simulink model "ParkAssist_Scenario002_cs"  (R2014b)
settings: Solver=ode5  SolverMode=SingleTasking  StartTime=0.0  StopTime=100  FixedStep=1/100  RelTol=1e-3
PreLoadFcn:
  | mbxruntime.callbacks.PreLoadFcn(bdroot);
  | check_NUTS_defined;
  | 
  | assignin('base',['model_closed_' bdroot],false);
  | addpath('../includes_AP');
PostLoadFcn:
  | mbxruntime.callbacks.PostLoadFcn(bdroot);
  | 
  | AP_PlotSpeed;
  | Sim_Stop();
InitFcn:
  | mbxruntime.callbacks.InitFcn(bdroot);
StartFcn:
  | mbxruntime.callbacks.StartFcn(bdroot);
StopFcn:
  | Sim_Stop();
  | 
  | mbxruntime.callbacks.StopFcn(bdroot);
model workspace: external: MAT-File .\ParkAssist_Scenario002_cs_hws.mat (data not in the file)
undefined symbols (not defined in the file or in its folder): mbxruntime, tabledata, warningInitialVelocity, x0
undefined symbols (not defined in the file): ParkAssist_Scenario002_cs_002fddfe84a374e6, ParkAssist_Scenario002_cs_01094a893a7092b9, ParkAssist_Scenario002_cs_02c2e05763b93088, ParkAssist_Scenario002_cs_032149ae54ddfcd1, ParkAssist_Scenario002_cs_03734bce5661314c, ParkAssist_Scenario002_cs_04091ed9282bd749, ParkAssist_Scenario002_cs_068635de1ad515a4, ParkAssist_Scenario002_cs_08968b565ab05e4d, ParkAssist_Scenario002_cs_08eaa26dcd990c9f, ParkAssist_Scenario002_cs_0a721129d3af9f72, ParkAssist_Scenario002_cs_0c5b0314074f54f3, ParkAssist_Scenario002_cs_0e48d515abeb5eec, ParkAssist_Scenario002_cs_1024d8e6ed1cbdcd, ParkAssist_Scenario002_cs_1193d522b107ebab, ParkAssist_Scenario002_cs_11dc16d46c17a7bf, ParkAssist_Scenario002_cs_13631b53806ed88f, ParkAssist_Scenario002_cs_155b57131b5ca1b3, ParkAssist_Scenario002_cs_1a68a29dae7c954c, ParkAssist_Scenario002_cs_1e925263f9fbaeb5, ParkAssist_Scenario002_cs_2102ebaddaee4634, ParkAssist_Scenario002_cs_242d7930853a635b, ParkAssist_Scenario002_cs_26123a651f74a75d, ParkAssist_Scenario002_cs_27077c166553ac4d, ParkAssist_Scenario002_cs_2775446e3f6a532e, ParkAssist_Scenario002_cs_29e1fcc85129d061, ParkAssist_Scenario002_cs_2c6c606bb8eb7e2a, ParkAssist_Scenario002_cs_2f026f6d085d63d4, ParkAssist_Scenario002_cs_2f66cf02f0c1fb02, ParkAssist_Scenario002_cs_2f7abfb8e98983ca, ParkAssist_Scenario002_cs_305144d476c37e1c, ParkAssist_Scenario002_cs_31c4862b0e1d31d2, ParkAssist_Scenario002_cs_3367812933b7aec5, ParkAssist_Scenario002_cs_338ceb4af5dab20a, ParkAssist_Scenario002_cs_359ca59699e4676c, ParkAssist_Scenario002_cs_374ade2de845ad31, ParkAssist_Scenario002_cs_390ab82ad2c54c91, ParkAssist_Scenario002_cs_391805fec31feab6, ParkAssist_Scenario002_cs_3974aed4b8055855, ParkAssist_Scenario002_cs_3a445c73fa984851, ParkAssist_Scenario002_cs_3a54967829cb62c8, ParkAssist_Scenario002_cs_3a60f4e734f7afb5, ParkAssist_Scenario002_cs_3bf2e9c0bde84b70, ParkAssist_Scenario002_cs_3c27f6f01aa99d37, ParkAssist_Scenario002_cs_3cc4b302268f6896, ParkAssist_Scenario002_cs_40419caba47c1546, ParkAssist_Scenario002_cs_42136abd911dac1d, ParkAssist_Scenario002_cs_44b760977392c607, ParkAssist_Scenario002_cs_470135ef0e52cc5f, ParkAssist_Scenario002_cs_48ebb83f5faed864, ParkAssist_Scenario002_cs_4a04bdc7976b10a4, ParkAssist_Scenario002_cs_4b414fc30cdb2355, ParkAssist_Scenario002_cs_4e3c7ad0309ae8ef, ParkAssist_Scenario002_cs_4f1cb442d755f69c, ParkAssist_Scenario002_cs_52f490d0aa621cbf, ParkAssist_Scenario002_cs_53df9d722ee02dea, ParkAssist_Scenario002_cs_5719a2c72af27d7c, ParkAssist_Scenario002_cs_575bfb9c514fb17e, ParkAssist_Scenario002_cs_588d2ca56dde3768, ParkAssist_Scenario002_cs_58ef6c537dd8a6a1, ParkAssist_Scenario002_cs_592f78d63a6470cd ... (+97)
libraries: PreScanUsefulBlocks x57, simulink x55, PreScanSimulinkLibrary x54, simulink_extras x6
(part 2 of 15)

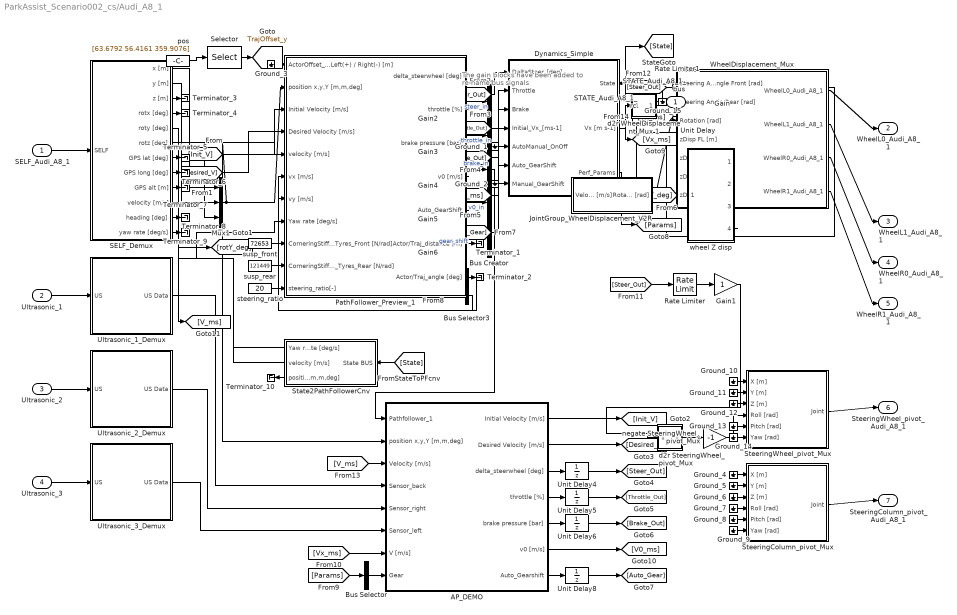
== system ParkAssist_Scenario002_cs/Audi_A8_1 ==
  note: The gain blocks have been added
      | to re-name bus signals
  SELF_Audi_A8_1 : Inport  Tag=inport/SelfPort  OutDataTypeStr=Bus: PRESCAN_SELFSENSORDATA  PortDimensions=1  SampleTime=1/100  BusOutputAsStruct=on
  Ultrasonic_1 : Inport  Tag=inport/UltraSonic  Port=2  OutDataTypeStr=Bus: PRESCAN_SCANNERSENSOR_MESSAGE  PortDimensions=1  SampleTime=1/20  BusOutputAsStruct=on
  Ultrasonic_2 : Inport  Tag=inport/UltraSonic  Port=3  OutDataTypeStr=Bus: PRESCAN_SCANNERSENSOR_MESSAGE  PortDimensions=1  SampleTime=1/20  BusOutputAsStruct=on
  Ultrasonic_3 : Inport  Tag=inport/UltraSonic  Port=4  OutDataTypeStr=Bus: PRESCAN_SCANNERSENSOR_MESSAGE  PortDimensions=1  SampleTime=1/20  BusOutputAsStruct=on
  AP_DEMO : Subsystem  mask(Park Assist System Mask){B_Length=5.21, B_Width=2.01, l=2.94, b=1.77, p1=1.28, p2=0.99, w=1.61, phi_max=25, SteerRatio=20, S_Range=6, S_XOffset=3.245, S_YOffset=0.950, Lmin_bay=3, offset_parallel=0.2}
      mask prompts: B_Length "Body length [m]"; B_Width "Body width [m]"; l "Wheelbase [m]"; b "Distance to the back wheel from cars center of gravity b [m]"; p1 "Rear overhang [m]"; p2 "Front overhang [m]"; w "Rear track tire width [m]"; phi_max "Max wheel angle [deg]"; SteerRatio "Steering Ratio [-]"; S_Range "Search Sensor Range [m]"; S_XOffset "Search Sensor X Offset [m]"; S_YOffset "Search Sensor Y Offset [m]"; Lmin_bay "Minimum bay parking space [m]"; offset_parallel "Parallel Parking Offset [m]"
      mask help: PreScan Experiment and Park Assist System parameters
      mask init:
      | SampleTime = str2num(get_param(bdroot,'FixedStep'));
      | DisplayFreq = 10; RadarFreq = DisplayFreq; IntDelay = (1/SampleTime)/DisplayFreq;
      | PathName = gcs;
      | R1 = l/sin(phi_max/180*pi);
      | R2 = sqrt(R1^2-l^2)-w/2;
      | R3 = sqrt((R2+w)^2+(l+p2)^2);
      | Lmin_parallel = p1+sqrt(R3^2-R2^2)+offset_parallel;
      mask Help: eval('openHelp(1136)')
  Bus Creator : BusCreator  Inputs=5
  Bus Selector : BusSelector  OutputSignals=Gear_[-]  OutputAsBus=on
  Bus Selector3 : BusSelector  OutputSignals=vx_[ms-1],vy_[ms-1]
  Dynamics_Simple : Subsystem  Tag=Simple_Vehicle_Dynamics  mask(PreScan Block: Simple Dynamics){TimeStep=1/100, ComputationMode=Continuous_Time, initialX=ParkAssist_Scenario002_cs_Audi_A8_1_Dynamics_Simple_initialX, initialY=ParkAssist_Scenario002_cs_Audi_A8_1_Dynamics_Simple_initialY, initialZ=ParkAssist_Scenario002_cs_Audi_A8_1_Dynamics_Simple_initialZ, initialRoll=ParkAssist_Scenario002_cs_Audi_A8_1_Dynamics_Simple_initialRoll, initialPitch=ParkAssist_Scenario002_cs_fbe23693a5827001, initialYaw=ParkAssist_Scenario002_cs_Audi_A8_1_Dynamics_Simple_initialYaw}
      mask prompts: TimeStep "Auto assigned: Time Step [s]"; ComputationMode "Computation mode:"; initialX "Ini x-position VEHICLE wrt GLOBAL axis system [m]"; initialY "Ini y-position VEHICLE wrt GLOBAL axis system [m]"; initialZ "Ini z-position VEHICLE wrt GLOBAL axis system [m]"; initialRoll "Ini roll-angle BODY wrt VEHICLE axis system [deg]"; initialPitch "Ini pitch-angle BODY wrt VEHICLE axis system [deg]"; initialYaw "Ini yaw-angle VEHICLE wrt GLOBAL axis system [deg]"
      mask help:
      | The Simple Dynamics Model is selected in the GUI to simulate vehicle dynamics behavior.
      |
      | The Simple Dynamics Model is completely open to the user. The parameters of this model can be set in the Simple Dynamics dialog in the GUI.
      |
      | For more information, please click Help.
      mask init:
      | p = SimpleDyn_pars;
      settings: DeleteFcn=PreScanBlockDeleteFcn;
      mask Help: eval('openHelp(220)')
      mask Display:
      | image(imread('SimpleDyn.png'))
      | port_label('input', 1, '{\delta}_S_t_ _e_e_r [deg]','texmode','on')
      | port_label('input', 2, 'Throttle [%]')
      | port_label('input', 3, 'Brake Pres [bar]')
      | port_label('input', 4, 'V_0 [ms-1]','texmode','on')
      | port_label('input', 5, 'Auto=[0]/Manual=[1]')
      | port_label('input', 6, 'Auto_GearShift')
      | port_label('input', 7, 'Manual_GearShift')
      | port_label('output', 1, 'State')
      | port_label('output', 2, 'Vx [ms-1]')
      | port_label('output', 3, 'Perf Params')
  Gain : Gain  Gain=1/20
  Gain{1..6} (6 alike) : Gain
  Ground_{1..15} (15 alike) : Ground
  JointGroup_WheelDisplacement_V2R : Subsystem  Tag=mux/Wheels  mask(PreScan Velocity to Wheel Angle Block:){TimeStep=1/100, TireRadius=0.34}
      mask prompts: TimeStep "Auto Assigned: Time Step [s]"; TireRadius "Tire Radius [m]"
      settings: DeleteFcn=PreScanBlockDeleteFcn;
      mask Display: disp('Velocity\nto\nWheelAngle')
  Mux1 : Mux  Inputs=3
  PathFollower_Preview_1 : Subsystem  Tag=PathFollower_Preview  mask(PreScan Block: Path Follower with Preview){LongCtrl_P=20, LongCtrl_I=0.3, LongCtrl_D=3.065, LongCtrl_AWU=1, LongCtrlDefault_P=20, LongCtrlDefault_I=0.3, LongCtrlDefault_D=3.065, LongCtrlDefault_AWU=1, PathUniqueID=ParkAssist_Scenario002_cs_d6af5f6999fe6828, mass=1820, Jzz=3746, length_a=1.17, length_l=2.94, Angle_Max_SteeringWheel=500, PreviewTime=1, DelayTime=0.1, LowSpeedLimit=20, MaxSteeringRate=1200, CSSampleTime=1/100, PFIntegrationFrequency=100}
      mask prompts: LongCtrl_P "Longitudinal Controller P"; LongCtrl_I "Longitudinal Controller I"; LongCtrl_D "Longitudinal Controller D"; LongCtrl_AWU "Longitudinal Controller AWU"; PathUniqueID "Path Unique ID"; mass "Mass vehicle total [kg]"; Jzz "Inertia vehicle around yaw axis [kg m2]"; length_a "Distance between COG and front axle [m]"; length_l "Length of wheelbase [m]"; Angle_Max_SteeringWheel "Maximum steering wheel angle [deg]"; PreviewTime "Preview time [s]"; DelayTime "Delay time [s]"; LowSpeedLimit "Low-speed limit [km/h]"; MaxSteeringRate "Maximum steering wheel angle rate [deg/s]"; CSSampleTime "Compilation Sheet sample time [s]"; PFIntegrationFrequency "Lateral controller frequency [Hz]"
      mask help:
      | The Path Follower Model is selected in the GUI to simulate driver behavior.
      |
      | For more information, please click Help.
      mask init:
      | RefreshCounter = max(floor((1/CSSampleTime) / (PFIntegrationFrequency)), 1);
      | PathFollowerBlockPath = gcb;
      mask Help: eval('openHelp(233)')
      mask DialogControl Control2 Prompt: Reset PID parameters
      mask DialogControl Control2 Callback:
      | LongCtrlDefault_P = get_param(gcb,'LongCtrlDefault_P');
      | set_param(gcb,'LongCtrl_P',LongCtrlDefault_P);
      | 
      | LongCtrlDefault_I = get_param(gcb,'LongCtrlDefault_I');
      | set_param(gcb,'LongCtrl_I',LongCtrlDefault_I);
      | 
      | LongCtrlDefault_D = get_param(gcb,'LongCtrlDefault_D');
      | set_param(gcb,'LongCtrl_D',LongCtrlDefault_D);
      | 
      | LongCtrlDefault_AWU = get_param(gcb,'LongCtrlDefault_AWU');
      | set_param(gcb,'LongCtrl_AWU',LongCtrlDefault_AWU);
  Rate Limiter : RateLimiter  RisingSlewLimit=500  FallingSlewLimit=-500  SampleTimeMode=inherited
  Rate Limiter1 : RateLimiter  RisingSlewLimit=500  FallingSlewLimit=-500  SampleTimeMode=inherited
  SELF_Demux : Subsystem  Tag=demux/SelfPort  mask(PreScan Demux Block:){}
      mask help:
      | The SELF port shows (state) information of the actor itself. The outputs are position in the experiment's axis system and the GPS coordinates, and the object's absolute velocity and compass heading.
      |
      | For more information, please click Help.
      settings: DeleteFcn=PreScanBlockDeleteFcn;
      mask Help: eval('openHelp(462)')
      mask Display:
      | port_label('output',1,'x [m]')
      | port_label('output',2,'y [m]')
      | port_label('output',3,'z [m]','texmode','on')
      | port_label('output',4,'Rotx [deg]','texmode','on')
      | port_label('output',5,'Roty [deg]','texmode','on')
      | port_label('output',6,'Rotz [deg]','texmode','on')
      | port_label('output',7,'GPS lat [deg]','texmode','on')
      | port_label('output',8,'GPS long [deg]','texmode','on')
      | port_label('output',9,'GPS alt [m]','texmode','on')
      | port_label('output',10,'Velocity [m/s]')
      | port_label('output',11,'Heading [deg]')
      | port_label('output',12,'Yaw rate [deg/s]')
  STATE_Audi_A8_1_rc : RateTransition  Tag=mux_rc/StatePort  OutPortSampleTimeOpt=Inherit
  Selector : Selector  InputPortWidth=3  Indices=[2]
  State2PathFollowerCnv : Subsystem  Tag=State2PFConnection/cnv
  SteeringColumn_pivot_Mux : Subsystem  Tag=mux/Joint  mask(PreScan Mux Block){DisplayName=SteeringColumn}
      mask prompts: DisplayName "Display Name"
      mask help:
      | This block simulates a generic joint used for generic models. This joint can be enabled/disabled from the GUI.
      |
      | For more information, please click Help.
      settings: DeleteFcn=PreScanBlockDeleteFcn;
      mask Help: eval('openHelp(254)')
  SteeringWheel_pivot_Mux : Subsystem  Tag=mux/Joint  mask(PreScan Mux Block){DisplayName=SteeringWheel}
      mask prompts: DisplayName "Display Name"
      mask help:
      | This block simulates a generic joint used for generic models. This joint can be enabled/disabled from the GUI.
      |
      | For more information, please click Help.
      settings: DeleteFcn=PreScanBlockDeleteFcn;
      mask Help: eval('openHelp(254)')
  Terminator_{1..10} (10 alike) : Terminator
  Ultrasonic_1_Demux : Subsystem  Tag=demux/Lidar  mask(PreScan Demux Block: UltraSonic){MAXMESSAGES=1}
      mask prompts: MAXMESSAGES "Number Of Objects"
      mask help:
      | The UltraSonic Sensor is a scanner device used to detect obstacles like cars, motor cycles, and pedestrians.
      |
      | For more information, please click Help.
      settings: DeleteFcn=PreScanBlockDeleteFcn;
      mask Help: eval('openHelp(1465)')
      mask Display:
      | port_label('input',1,'US')
      | port_label('output',1,'US Data')
  Ultrasonic_2_Demux : Subsystem  Tag=demux/Lidar  mask(PreScan Demux Block: UltraSonic){MAXMESSAGES=1}
      mask prompts: MAXMESSAGES "Number Of Objects"
      mask help:
      | The UltraSonic Sensor is a scanner device used to detect obstacles like cars, motor cycles, and pedestrians.
      |
      | For more information, please click Help.
      settings: DeleteFcn=PreScanBlockDeleteFcn;
      mask Help: eval('openHelp(1465)')
      mask Display:
      | port_label('input',1,'US')
      | port_label('output',1,'US Data')
  Ultrasonic_3_Demux : Subsystem  Tag=demux/Lidar  mask(PreScan Demux Block: UltraSonic){MAXMESSAGES=1}
      mask prompts: MAXMESSAGES "Number Of Objects"
      mask help:
      | The UltraSonic Sensor is a scanner device used to detect obstacles like cars, motor cycles, and pedestrians.
      |
      | For more information, please click Help.
      settings: DeleteFcn=PreScanBlockDeleteFcn;
      mask Help: eval('openHelp(1465)')
      mask Display:
      | port_label('input',1,'US')
      | port_label('output',1,'US Data')
  Unit Delay{,4..6,8} (5 alike) : UnitDelay  SampleTime=-1
  WheelDisplacement_Mux : Subsystem  Tag=mux/JointGroup  mask(JointGroup){}
      mask help:
      | The JointGroup allows to control several Joints in one go, as defined for this particular model.
      | For more information, look in the PreScan manual in the section "Model Preparation Tool" -> "Joint Groups"
      |
      | For more information on the Joints simulink interface, press Help.
      mask Help: eval('openHelp(254)')
  d2r SteeringWheel_pivot_Mux : Subsystem  mask(DegreesToRadians){}
      mask help: SimulinkBlocks:simulink_extras:DegreesToRadians_MD
      mask Help: web([docroot '/simulink/ref_extras/degreestoradians.html'])
      mask Display: disp('D2R')
  d2r WheelDisplacement_Mux 1 : Subsystem  mask(DegreesToRadians){}
      mask help: SimulinkBlocks:simulink_extras:DegreesToRadians_MD
      mask Help: web([docroot '/simulink/ref_extras/degreestoradians.html'])
      mask Display: disp('D2R')
  negate SteeringWheel_pivot_Mux : Gain  Gain=-1
  pos : Constant  Tag=pos  Value=[63.6792 56.4161 359.9076]
  steering_ratio : Constant  Tag=steering_ratio  Value=20
  susp_front : Constant  Tag=susp_front  Value=72653
  susp_rear : Constant  Tag=susp_rear  Value=121449
  wheel Z disp : Subsystem  mask(Simple Dynamics parameters){a=1.20, b=1.45}
      mask prompts: a "Distance to the front wheel from cars center of gravity a [m]"; b "Distance to the back wheel from cars center of gravity b [m]"
  STATE_Audi_A8_1_bus : Outport  Tag=outport/StatePort  OutDataTypeStr=Bus: PRESCAN_STATEACTUATORDATA  PortDimensions=1  SampleTime=1/100
  WheelL0_Audi_A8_1 : Outport  Tag=outport/JointActuator  Port=2  OutDataTypeStr=Bus: PRESCAN_POSE_DATA  SampleTime=1/100
  WheelL1_Audi_A8_1 : Outport  Tag=outport/JointActuator  Port=3  OutDataTypeStr=Bus: PRESCAN_POSE_DATA  SampleTime=1/100
  WheelR0_Audi_A8_1 : Outport  Tag=outport/JointActuator  Port=4  OutDataTypeStr=Bus: PRESCAN_POSE_DATA  SampleTime=1/100
  WheelR1_Audi_A8_1 : Outport  Tag=outport/JointActuator  Port=5  OutDataTypeStr=Bus: PRESCAN_POSE_DATA  SampleTime=1/100
  SteeringWheel_pivot_Audi_A8_1 : Outport  Tag=outport/JointActuator  Port=6  OutDataTypeStr=Bus: PRESCAN_POSE_DATA  SampleTime=1/100
  SteeringColumn_pivot_Audi_A8_1 : Outport  Tag=outport/JointActuator  Port=7  OutDataTypeStr=Bus: PRESCAN_POSE_DATA  SampleTime=1/100
  tag scope: TrajOffset_y=global
  wires:
  AP_DEMO/1(Initial Velocity [m/s]) -> [Init_V]
  AP_DEMO/2(Desired Velocity [m/s]) -> [Desired_V]
  AP_DEMO/3(delta_steerwheel [deg]) -> Unit Delay4/1
  Unit Delay4/1 -> [Steer_Out]
  AP_DEMO/4(throttle [%]) -> Unit Delay5/1
  Unit Delay5/1 -> [Throttle_Out]
  AP_DEMO/5(brake pressure [bar]) -> Unit Delay6/1
  Unit Delay6/1 -> [Brake_Out]
  AP_DEMO/6(v0 [m/s]) -> [V0_ms]
  AP_DEMO/7(Auto_Gearshift) -> Unit Delay8/1
  Unit Delay8/1 -> [Auto_Gear]
  Bus Creator/1 -> AP_DEMO/1(Pathfollower_1)
  Gain2/1 -> Bus Creator/1  "steer_in"
  Gain3/1 -> Bus Creator/2  "throttle_in"
  Gain4/1 -> Bus Creator/3  "brake_in"
  Gain5/1 -> Bus Creator/4  "v0_in"
  Gain6/1 -> Bus Creator/5  "gear_shift"
  Mux1/1 -> AP_DEMO/2(position x,y,Y [m,m,deg]), PathFollower_Preview_1/2(position x,y,Y [m,m,deg])
  [V_ms] -> AP_DEMO/3(Velocity [m/s])
  [Vx_ms] -> AP_DEMO/7(V [m/s])
  Bus Selector/1 -> AP_DEMO/8(Gear)
  [Params] -> Bus Selector/1
  PathFollower_Preview_1/1(delta_steerwheel [deg]) -> Gain2/1
  PathFollower_Preview_1/2(throttle [%]) -> Gain3/1
  PathFollower_Preview_1/3(brake pressure [bar]) -> Gain4/1
  PathFollower_Preview_1/4(v0 [m/s]) -> Gain5/1
  PathFollower_Preview_1/5(Auto_GearShift) -> Gain6/1
  SELF_Demux/1(x [m]) -> Mux1/1
  SELF_Demux/2(y [m]) -> Mux1/2
  SELF_Demux/6(rotz [deg]) -> Mux1/3
  Ultrasonic_1_Demux/1(US Data) -> AP_DEMO/4(Sensor_back)
  Ultrasonic_2_Demux/1(US Data) -> AP_DEMO/5(Sensor_right)
  Ultrasonic_3_Demux/1(US Data) -> AP_DEMO/6(Sensor_left)
  [Params] -> Bus Selector3/1
  Bus Selector3/1 -> PathFollower_Preview_1/6(vx [m/s])
  Bus Selector3/2 -> PathFollower_Preview_1/7(vy [m/s])
  [Init_V] -> PathFollower_Preview_1/3(Initial Velocity [m/s])
  [Desired_V] -> PathFollower_Preview_1/4(Desired Velocity [m/s])
  [Steer_Out] -> Rate Limiter/1
  Rate Limiter/1 -> Gain1/1
  Gain1/1 -> d2r SteeringWheel_pivot_Mux/1(Degrees in)
  d2r SteeringWheel_pivot_Mux/1(Radians out) -> negate SteeringWheel_pivot_Mux/1
  negate SteeringWheel_pivot_Mux/1 -> SteeringWheel_pivot_Mux/4(Roll [rad])
  [Steer_Out] -> Rate Limiter1/1
  Rate Limiter1/1 -> Gain/1
  Gain/1 -> d2r WheelDisplacement_Mux 1/1(Degrees in)
  d2r WheelDisplacement_Mux 1/1(Radians out) -> WheelDisplacement_Mux/1(Steering Angle Front [rad])
  [Vx_ms] -> Unit Delay/1
  Unit Delay/1 -> JointGroup_WheelDisplacement_V2R/1(Velocity [m/s])
  [Steer_Out] -> Dynamics_Simple/1(DeltaSteer_[deg])
  [Throttle_Out] -> Dynamics_Simple/2(Throttle)
  [Brake_Out] -> Dynamics_Simple/3(Brake)
  [V0_ms] -> Dynamics_Simple/4(Initial_Vx_[ms-1])
  [rotY_deg] -> wheel Z disp/1(rotY [deg])
  wheel Z disp/1(zDisp FL [m]) -> WheelDisplacement_Mux/4(zDisp FL [m])
  wheel Z disp/2(zDisp FR [m]) -> WheelDisplacement_Mux/5(zDisp FR [m])
  wheel Z disp/3(zDisp RL [m]) -> WheelDisplacement_Mux/6(zDisp RL [m])
  wheel Z disp/4(zDisp RR [m]) -> WheelDisplacement_Mux/7(zDisp RR [m])
  [Auto_Gear] -> Dynamics_Simple/6(Auto_GearShift)
  Selector/1 -> [TrajOffset_y]
  pos/1 -> Selector/1
  SELF_Demux/5(roty [deg]) -> [rotY_deg]
  SELF_Demux/10(velocity [m/s]) -> [V_ms]
  Dynamics_Simple/3(Perf_Params) -> [Params]
  Dynamics_Simple/2(Vx [m s-1]) -> [Vx_ms]
  Dynamics_Simple/1(State) -> STATE_Audi_A8_1_rc/1, [State]
  STATE_Audi_A8_1_rc/1 -> STATE_Audi_A8_1_bus/1
  SELF_Audi_A8_1/1 -> SELF_Demux/1(SELF)
  Ultrasonic_1/1 -> Ultrasonic_1_Demux/1(US)
  Ultrasonic_2/1 -> Ultrasonic_2_Demux/1(US)
  Ultrasonic_3/1 -> Ultrasonic_3_Demux/1(US)
  WheelDisplacement_Mux/1(WheelL0_Audi_A8_1) -> WheelL0_Audi_A8_1/1
  WheelDisplacement_Mux/2(WheelL1_Audi_A8_1) -> WheelL1_Audi_A8_1/1
  WheelDisplacement_Mux/3(WheelR0_Audi_A8_1) -> WheelR0_Audi_A8_1/1
  WheelDisplacement_Mux/4(WheelR1_Audi_A8_1) -> WheelR1_Audi_A8_1/1
  JointGroup_WheelDisplacement_V2R/1(Rotation [rad]) -> WheelDisplacement_Mux/3(Rotation [rad])
  SteeringWheel_pivot_Mux/1(Joint) -> SteeringWheel_pivot_Audi_A8_1/1
  SteeringColumn_pivot_Mux/1(Joint) -> SteeringColumn_pivot_Audi_A8_1/1
  susp_front/1 -> PathFollower_Preview_1/9(CorneringStiffness_Tyres_Front [N/rad])
  susp_rear/1 -> PathFollower_Preview_1/10(CorneringStiffness_Tyres_Rear [N/rad])
  steering_ratio/1 -> PathFollower_Preview_1/11(steering_ratio[-])
  [State] -> State2PathFollowerCnv/1(State BUS)
  State2PathFollowerCnv/1(Yaw rate [deg/s]) -> PathFollower_Preview_1/8(Yaw rate [deg/s])
  State2PathFollowerCnv/2(velocity [m/s]) -> PathFollower_Preview_1/5(velocity [m/s])
  Ground_1/1 -> Dynamics_Simple/5(AutoManual_OnOff)
  Ground_2/1 -> Dynamics_Simple/7(Manual_GearShift)
  Ground_3/1 -> PathFollower_Preview_1/1(ActorOffset_Left(+) / Right(-) [m])
  PathFollower_Preview_1/6(Actor/Traj_distance [m]) -> Terminator_1/1
  PathFollower_Preview_1/7(Actor/Traj_angle [deg]) -> Terminator_2/1
  SELF_Demux/3(z [m]) -> Terminator_3/1
  SELF_Demux/4(rotx [deg]) -> Terminator_4/1
  SELF_Demux/7(GPS lat [deg]) -> Terminator_5/1
  SELF_Demux/8(GPS long [deg]) -> Terminator_6/1
  SELF_Demux/9(GPS alt [m]) -> Terminator_7/1
  SELF_Demux/11(heading [deg]) -> Terminator_8/1
  SELF_Demux/12(yaw rate [deg/s]) -> Terminator_9/1
  State2PathFollowerCnv/3(position x,y,Y [m,m,deg]) -> Terminator_10/1
  Ground_4/1 -> SteeringColumn_pivot_Mux/1(X [m])
  Ground_5/1 -> SteeringColumn_pivot_Mux/2(Y [m])
  Ground_6/1 -> SteeringColumn_pivot_Mux/3(Z [m])
  Ground_7/1 -> SteeringColumn_pivot_Mux/4(Roll [rad])
  Ground_8/1 -> SteeringColumn_pivot_Mux/5(Pitch [rad])
  Ground_9/1 -> SteeringColumn_pivot_Mux/6(Yaw [rad])
  Ground_10/1 -> SteeringWheel_pivot_Mux/1(X [m])
  Ground_11/1 -> SteeringWheel_pivot_Mux/2(Y [m])
  Ground_12/1 -> SteeringWheel_pivot_Mux/3(Z [m])
  Ground_13/1 -> SteeringWheel_pivot_Mux/5(Pitch [rad])
  Ground_14/1 -> SteeringWheel_pivot_Mux/6(Yaw [rad])
  Ground_15/1 -> WheelDisplacement_Mux/2(Steering Angle Rear [rad])

== system ParkAssist_Scenario002_cs/Audi_A8_10 ==
  SELF_Audi_A8_10 : Inport  Tag=inport/SelfPort  OutDataTypeStr=Bus: PRESCAN_SELFSENSORDATA  PortDimensions=1  SampleTime=1/100  BusOutputAsStruct=on
  ColorRegion_Exterior_color : Constant  Tag=VisuLightConst  Value=[25 25 112]
  Dynamics_Empty : Subsystem  Tag=Dynamics_Empty
      mask Help: eval('openHelp(202)')
      mask Display: port_label('output', 1, 'State');text(0,0,' Empty\n')
  SELF_Demux : Subsystem  Tag=demux/SelfPort  mask(PreScan Demux Block:){}
      mask help:
      | The SELF port shows (state) information of the actor itself. The outputs are position in the experiment's axis system and the GPS coordinates, and the object's absolute velocity and compass heading.
      |
      | For more information, please click Help.
      settings: DeleteFcn=PreScanBlockDeleteFcn;
      mask Help: eval('openHelp(462)')
      mask Display:
      | port_label('output',1,'x [m]')
      | port_label('output',2,'y [m]')
      | port_label('output',3,'z [m]','texmode','on')
      | port_label('output',4,'Rotx [deg]','texmode','on')
      | port_label('output',5,'Roty [deg]','texmode','on')
      | port_label('output',6,'Rotz [deg]','texmode','on')
      | port_label('output',7,'GPS lat [deg]','texmode','on')
      | port_label('output',8,'GPS long [deg]','texmode','on')
      | port_label('output',9,'GPS alt [m]','texmode','on')
      | port_label('output',10,'Velocity [m/s]')
      | port_label('output',11,'Heading [deg]')
      | port_label('output',12,'Yaw rate [deg/s]')
  STATE_Audi_A8_10_rc : RateTransition  Tag=mux_rc/StatePort  OutPortSampleTimeOpt=Inherit
  Terminator_{1..12} (12 alike) : Terminator
  VISUColorRegion_Exterior_Mux : Subsystem  Tag=mux/MuxColorRegion  LoadFcn=load PrescanColorData  mask(PreScan User Interface: VisuTextureColor){}
      mask help:
      | The VisuTextureColor block provides a way to adapt the color of a vehicle.
      |
      | For more information, please click Help.
      settings: DeleteFcn=PreScanBlockDeleteFcn;
      mask Help: eval('openHelp(230)')
  STATE_Audi_A8_10_bus : Outport  Tag=outport/StatePort  OutDataTypeStr=Bus: PRESCAN_STATEACTUATORDATA  PortDimensions=1  SampleTime=1/100
  VISUColorRegion_Exterior_Audi_A8_10 : Outport  Tag=outport/ColorRegion  Port=2  OutDataTypeStr=Bus: PRESCAN_COLOR_DATA  PortDimensions=1  SampleTime=1/100
  wires:
  STATE_Audi_A8_10_rc/1 -> STATE_Audi_A8_10_bus/1
  SELF_Audi_A8_10/1 -> SELF_Demux/1(SELF)
  VISUColorRegion_Exterior_Mux/1(ColorRegion) -> VISUColorRegion_Exterior_Audi_A8_10/1
  ColorRegion_Exterior_color/1 -> VISUColorRegion_Exterior_Mux/1(RGB [-,-,-])
  Dynamics_Empty/1(State) -> STATE_Audi_A8_10_rc/1
  SELF_Demux/1(x [m]) -> Terminator_1/1
  SELF_Demux/2(y [m]) -> Terminator_2/1
  SELF_Demux/3(z [m]) -> Terminator_3/1
  SELF_Demux/4(rotx [deg]) -> Terminator_4/1
  SELF_Demux/5(roty [deg]) -> Terminator_5/1
  SELF_Demux/6(rotz [deg]) -> Terminator_6/1
  SELF_Demux/7(GPS lat [deg]) -> Terminator_7/1
  SELF_Demux/8(GPS long [deg]) -> Terminator_8/1
  SELF_Demux/9(GPS alt [m]) -> Terminator_9/1
  SELF_Demux/10(velocity [m/s]) -> Terminator_10/1
  SELF_Demux/11(heading [deg]) -> Terminator_11/1
  SELF_Demux/12(yaw rate [deg/s]) -> Terminator_12/1

== system ParkAssist_Scenario002_cs/Audi_A8_13 ==
  SELF_Audi_A8_13 : Inport  Tag=inport/SelfPort  OutDataTypeStr=Bus: PRESCAN_SELFSENSORDATA  PortDimensions=1  SampleTime=1/100  BusOutputAsStruct=on
  ColorRegion_Exterior_color : Constant  Tag=VisuLightConst  Value=[165 42 42]
  Dynamics_Empty : Subsystem  Tag=Dynamics_Empty
      mask Help: eval('openHelp(202)')
      mask Display: port_label('output', 1, 'State');text(0,0,' Empty\n')
  SELF_Demux : Subsystem  Tag=demux/SelfPort  mask(PreScan Demux Block:){}
      mask help:
      | The SELF port shows (state) information of the actor itself. The outputs are position in the experiment's axis system and the GPS coordinates, and the object's absolute velocity and compass heading.
      |
      | For more information, please click Help.
      settings: DeleteFcn=PreScanBlockDeleteFcn;
      mask Help: eval('openHelp(462)')
      mask Display:
      | port_label('output',1,'x [m]')
      | port_label('output',2,'y [m]')
      | port_label('output',3,'z [m]','texmode','on')
      | port_label('output',4,'Rotx [deg]','texmode','on')
      | port_label('output',5,'Roty [deg]','texmode','on')
      | port_label('output',6,'Rotz [deg]','texmode','on')
      | port_label('output',7,'GPS lat [deg]','texmode','on')
      | port_label('output',8,'GPS long [deg]','texmode','on')
      | port_label('output',9,'GPS alt [m]','texmode','on')
      | port_label('output',10,'Velocity [m/s]')
      | port_label('output',11,'Heading [deg]')
      | port_label('output',12,'Yaw rate [deg/s]')
  STATE_Audi_A8_13_rc : RateTransition  Tag=mux_rc/StatePort  OutPortSampleTimeOpt=Inherit
  Terminator_{1..12} (12 alike) : Terminator
  VISUColorRegion_Exterior_Mux : Subsystem  Tag=mux/MuxColorRegion  LoadFcn=load PrescanColorData  mask(PreScan User Interface: VisuTextureColor){}
      mask help:
      | The VisuTextureColor block provides a way to adapt the color of a vehicle.
      |
      | For more information, please click Help.
      settings: DeleteFcn=PreScanBlockDeleteFcn;
      mask Help: eval('openHelp(230)')
  STATE_Audi_A8_13_bus : Outport  Tag=outport/StatePort  OutDataTypeStr=Bus: PRESCAN_STATEACTUATORDATA  PortDimensions=1  SampleTime=1/100
  VISUColorRegion_Exterior_Audi_A8_13 : Outport  Tag=outport/ColorRegion  Port=2  OutDataTypeStr=Bus: PRESCAN_COLOR_DATA  PortDimensions=1  SampleTime=1/100
  wires:
  STATE_Audi_A8_13_rc/1 -> STATE_Audi_A8_13_bus/1
  SELF_Audi_A8_13/1 -> SELF_Demux/1(SELF)
  VISUColorRegion_Exterior_Mux/1(ColorRegion) -> VISUColorRegion_Exterior_Audi_A8_13/1
  ColorRegion_Exterior_color/1 -> VISUColorRegion_Exterior_Mux/1(RGB [-,-,-])
  Dynamics_Empty/1(State) -> STATE_Audi_A8_13_rc/1
  SELF_Demux/1(x [m]) -> Terminator_1/1
  SELF_Demux/2(y [m]) -> Terminator_2/1
  SELF_Demux/3(z [m]) -> Terminator_3/1
  SELF_Demux/4(rotx [deg]) -> Terminator_4/1
  SELF_Demux/5(roty [deg]) -> Terminator_5/1
  SELF_Demux/6(rotz [deg]) -> Terminator_6/1
  SELF_Demux/7(GPS lat [deg]) -> Terminator_7/1
  SELF_Demux/8(GPS long [deg]) -> Terminator_8/1
  SELF_Demux/9(GPS alt [m]) -> Terminator_9/1
  SELF_Demux/10(velocity [m/s]) -> Terminator_10/1
  SELF_Demux/11(heading [deg]) -> Terminator_11/1
  SELF_Demux/12(yaw rate [deg/s]) -> Terminator_12/1

== system ParkAssist_Scenario002_cs/Audi_A8_14 ==
  SELF_Audi_A8_14 : Inport  Tag=inport/SelfPort  OutDataTypeStr=Bus: PRESCAN_SELFSENSORDATA  PortDimensions=1  SampleTime=1/100  BusOutputAsStruct=on
  ColorRegion_Exterior_color : Constant  Tag=VisuLightConst  Value=[211 211 211]
  Dynamics_Empty : Subsystem  Tag=Dynamics_Empty
      mask Help: eval('openHelp(202)')
      mask Display: port_label('output', 1, 'State');text(0,0,' Empty\n')
  SELF_Demux : Subsystem  Tag=demux/SelfPort  mask(PreScan Demux Block:){}
      mask help:
      | The SELF port shows (state) information of the actor itself. The outputs are position in the experiment's axis system and the GPS coordinates, and the object's absolute velocity and compass heading.
      |
      | For more information, please click Help.
      settings: DeleteFcn=PreScanBlockDeleteFcn;
      mask Help: eval('openHelp(462)')
      mask Display:
      | port_label('output',1,'x [m]')
      | port_label('output',2,'y [m]')
      | port_label('output',3,'z [m]','texmode','on')
      | port_label('output',4,'Rotx [deg]','texmode','on')
      | port_label('output',5,'Roty [deg]','texmode','on')
      | port_label('output',6,'Rotz [deg]','texmode','on')
      | port_label('output',7,'GPS lat [deg]','texmode','on')
      | port_label('output',8,'GPS long [deg]','texmode','on')
      | port_label('output',9,'GPS alt [m]','texmode','on')
      | port_label('output',10,'Velocity [m/s]')
      | port_label('output',11,'Heading [deg]')
      | port_label('output',12,'Yaw rate [deg/s]')
  STATE_Audi_A8_14_rc : RateTransition  Tag=mux_rc/StatePort  OutPortSampleTimeOpt=Inherit
  Terminator_{1..12} (12 alike) : Terminator
  VISUColorRegion_Exterior_Mux : Subsystem  Tag=mux/MuxColorRegion  LoadFcn=load PrescanColorData  mask(PreScan User Interface: VisuTextureColor){}
      mask help:
      | The VisuTextureColor block provides a way to adapt the color of a vehicle.
      |
      | For more information, please click Help.
      settings: DeleteFcn=PreScanBlockDeleteFcn;
      mask Help: eval('openHelp(230)')
  STATE_Audi_A8_14_bus : Outport  Tag=outport/StatePort  OutDataTypeStr=Bus: PRESCAN_STATEACTUATORDATA  PortDimensions=1  SampleTime=1/100
  VISUColorRegion_Exterior_Audi_A8_14 : Outport  Tag=outport/ColorRegion  Port=2  OutDataTypeStr=Bus: PRESCAN_COLOR_DATA  PortDimensions=1  SampleTime=1/100
  wires:
  STATE_Audi_A8_14_rc/1 -> STATE_Audi_A8_14_bus/1
  SELF_Audi_A8_14/1 -> SELF_Demux/1(SELF)
  VISUColorRegion_Exterior_Mux/1(ColorRegion) -> VISUColorRegion_Exterior_Audi_A8_14/1
  ColorRegion_Exterior_color/1 -> VISUColorRegion_Exterior_Mux/1(RGB [-,-,-])
  Dynamics_Empty/1(State) -> STATE_Audi_A8_14_rc/1
  SELF_Demux/1(x [m]) -> Terminator_1/1
  SELF_Demux/2(y [m]) -> Terminator_2/1
  SELF_Demux/3(z [m]) -> Terminator_3/1
  SELF_Demux/4(rotx [deg]) -> Terminator_4/1
  SELF_Demux/5(roty [deg]) -> Terminator_5/1
  SELF_Demux/6(rotz [deg]) -> Terminator_6/1
  SELF_Demux/7(GPS lat [deg]) -> Terminator_7/1
  SELF_Demux/8(GPS long [deg]) -> Terminator_8/1
  SELF_Demux/9(GPS alt [m]) -> Terminator_9/1
  SELF_Demux/10(velocity [m/s]) -> Terminator_10/1
  SELF_Demux/11(heading [deg]) -> Terminator_11/1
  SELF_Demux/12(yaw rate [deg/s]) -> Terminator_12/1

== system ParkAssist_Scenario002_cs/Audi_A8_2 ==
  SELF_Audi_A8_2 : Inport  Tag=inport/SelfPort  OutDataTypeStr=Bus: PRESCAN_SELFSENSORDATA  PortDimensions=1  SampleTime=1/100  BusOutputAsStruct=on
  ColorRegion_Exterior_color : Constant  Tag=VisuLightConst  Value=[165 42 42]
  Dynamics_Empty : Subsystem  Tag=Dynamics_Empty
      mask Help: eval('openHelp(202)')
      mask Display: port_label('output', 1, 'State');text(0,0,' Empty\n')
  SELF_Demux : Subsystem  Tag=demux/SelfPort  mask(PreScan Demux Block:){}
      mask help:
      | The SELF port shows (state) information of the actor itself. The outputs are position in the experiment's axis system and the GPS coordinates, and the object's absolute velocity and compass heading.
      |
      | For more information, please click Help.
      settings: DeleteFcn=PreScanBlockDeleteFcn;
      mask Help: eval('openHelp(462)')
      mask Display:
      | port_label('output',1,'x [m]')
      | port_label('output',2,'y [m]')
      | port_label('output',3,'z [m]','texmode','on')
      | port_label('output',4,'Rotx [deg]','texmode','on')
      | port_label('output',5,'Roty [deg]','texmode','on')
      | port_label('output',6,'Rotz [deg]','texmode','on')
      | port_label('output',7,'GPS lat [deg]','texmode','on')
      | port_label('output',8,'GPS long [deg]','texmode','on')
      | port_label('output',9,'GPS alt [m]','texmode','on')
      | port_label('output',10,'Velocity [m/s]')
      | port_label('output',11,'Heading [deg]')
      | port_label('output',12,'Yaw rate [deg/s]')
  STATE_Audi_A8_2_rc : RateTransition  Tag=mux_rc/StatePort  OutPortSampleTimeOpt=Inherit
  Terminator_{1..12} (12 alike) : Terminator
  VISUColorRegion_Exterior_Mux : Subsystem  Tag=mux/MuxColorRegion  LoadFcn=load PrescanColorData  mask(PreScan User Interface: VisuTextureColor){}
      mask help:
      | The VisuTextureColor block provides a way to adapt the color of a vehicle.
      |
      | For more information, please click Help.
      settings: DeleteFcn=PreScanBlockDeleteFcn;
      mask Help: eval('openHelp(230)')
  STATE_Audi_A8_2_bus : Outport  Tag=outport/StatePort  OutDataTypeStr=Bus: PRESCAN_STATEACTUATORDATA  PortDimensions=1  SampleTime=1/100
  VISUColorRegion_Exterior_Audi_A8_2 : Outport  Tag=outport/ColorRegion  Port=2  OutDataTypeStr=Bus: PRESCAN_COLOR_DATA  PortDimensions=1  SampleTime=1/100
  wires:
  STATE_Audi_A8_2_rc/1 -> STATE_Audi_A8_2_bus/1
  SELF_Audi_A8_2/1 -> SELF_Demux/1(SELF)
  VISUColorRegion_Exterior_Mux/1(ColorRegion) -> VISUColorRegion_Exterior_Audi_A8_2/1
  ColorRegion_Exterior_color/1 -> VISUColorRegion_Exterior_Mux/1(RGB [-,-,-])
  Dynamics_Empty/1(State) -> STATE_Audi_A8_2_rc/1
  SELF_Demux/1(x [m]) -> Terminator_1/1
  SELF_Demux/2(y [m]) -> Terminator_2/1
  SELF_Demux/3(z [m]) -> Terminator_3/1
  SELF_Demux/4(rotx [deg]) -> Terminator_4/1
  SELF_Demux/5(roty [deg]) -> Terminator_5/1
  SELF_Demux/6(rotz [deg]) -> Terminator_6/1
  SELF_Demux/7(GPS lat [deg]) -> Terminator_7/1
  SELF_Demux/8(GPS long [deg]) -> Terminator_8/1
  SELF_Demux/9(GPS alt [m]) -> Terminator_9/1
  SELF_Demux/10(velocity [m/s]) -> Terminator_10/1
  SELF_Demux/11(heading [deg]) -> Terminator_11/1
  SELF_Demux/12(yaw rate [deg/s]) -> Terminator_12/1

== system ParkAssist_Scenario002_cs/Audi_A8_3 ==
  SELF_Audi_A8_3 : Inport  Tag=inport/SelfPort  OutDataTypeStr=Bus: PRESCAN_SELFSENSORDATA  PortDimensions=1  SampleTime=1/100  BusOutputAsStruct=on
  ColorRegion_Exterior_color : Constant  Tag=VisuLightConst  Value=[165 42 42]
  Dynamics_Empty : Subsystem  Tag=Dynamics_Empty
      mask Help: eval('openHelp(202)')
      mask Display: port_label('output', 1, 'State');text(0,0,' Empty\n')
  SELF_Demux : Subsystem  Tag=demux/SelfPort  mask(PreScan Demux Block:){}
      mask help:
      | The SELF port shows (state) information of the actor itself. The outputs are position in the experiment's axis system and the GPS coordinates, and the object's absolute velocity and compass heading.
      |
      | For more information, please click Help.
      settings: DeleteFcn=PreScanBlockDeleteFcn;
      mask Help: eval('openHelp(462)')
      mask Display:
      | port_label('output',1,'x [m]')
      | port_label('output',2,'y [m]')
      | port_label('output',3,'z [m]','texmode','on')
      | port_label('output',4,'Rotx [deg]','texmode','on')
      | port_label('output',5,'Roty [deg]','texmode','on')
      | port_label('output',6,'Rotz [deg]','texmode','on')
      | port_label('output',7,'GPS lat [deg]','texmode','on')
      | port_label('output',8,'GPS long [deg]','texmode','on')
      | port_label('output',9,'GPS alt [m]','texmode','on')
      | port_label('output',10,'Velocity [m/s]')
      | port_label('output',11,'Heading [deg]')
      | port_label('output',12,'Yaw rate [deg/s]')
  STATE_Audi_A8_3_rc : RateTransition  Tag=mux_rc/StatePort  OutPortSampleTimeOpt=Inherit
  Terminator_{1..12} (12 alike) : Terminator
  VISUColorRegion_Exterior_Mux : Subsystem  Tag=mux/MuxColorRegion  LoadFcn=load PrescanColorData  mask(PreScan User Interface: VisuTextureColor){}
      mask help:
      | The VisuTextureColor block provides a way to adapt the color of a vehicle.
      |
      | For more information, please click Help.
      settings: DeleteFcn=PreScanBlockDeleteFcn;
      mask Help: eval('openHelp(230)')
  STATE_Audi_A8_3_bus : Outport  Tag=outport/StatePort  OutDataTypeStr=Bus: PRESCAN_STATEACTUATORDATA  PortDimensions=1  SampleTime=1/100
  VISUColorRegion_Exterior_Audi_A8_3 : Outport  Tag=outport/ColorRegion  Port=2  OutDataTypeStr=Bus: PRESCAN_COLOR_DATA  PortDimensions=1  SampleTime=1/100
  wires:
  STATE_Audi_A8_3_rc/1 -> STATE_Audi_A8_3_bus/1
  SELF_Audi_A8_3/1 -> SELF_Demux/1(SELF)
  VISUColorRegion_Exterior_Mux/1(ColorRegion) -> VISUColorRegion_Exterior_Audi_A8_3/1
  ColorRegion_Exterior_color/1 -> VISUColorRegion_Exterior_Mux/1(RGB [-,-,-])
  Dynamics_Empty/1(State) -> STATE_Audi_A8_3_rc/1
  SELF_Demux/1(x [m]) -> Terminator_1/1
  SELF_Demux/2(y [m]) -> Terminator_2/1
  SELF_Demux/3(z [m]) -> Terminator_3/1
  SELF_Demux/4(rotx [deg]) -> Terminator_4/1
  SELF_Demux/5(roty [deg]) -> Terminator_5/1
  SELF_Demux/6(rotz [deg]) -> Terminator_6/1
  SELF_Demux/7(GPS lat [deg]) -> Terminator_7/1
  SELF_Demux/8(GPS long [deg]) -> Terminator_8/1
  SELF_Demux/9(GPS alt [m]) -> Terminator_9/1
  SELF_Demux/10(velocity [m/s]) -> Terminator_10/1
  SELF_Demux/11(heading [deg]) -> Terminator_11/1
  SELF_Demux/12(yaw rate [deg/s]) -> Terminator_12/1

== system ParkAssist_Scenario002_cs/Audi_A8_4 ==
  SELF_Audi_A8_4 : Inport  Tag=inport/SelfPort  OutDataTypeStr=Bus: PRESCAN_SELFSENSORDATA  PortDimensions=1  SampleTime=1/100  BusOutputAsStruct=on
  ColorRegion_Exterior_color : Constant  Tag=VisuLightConst  Value=[211 211 211]
  Dynamics_Empty : Subsystem  Tag=Dynamics_Empty
      mask Help: eval('openHelp(202)')
      mask Display: port_label('output', 1, 'State');text(0,0,' Empty\n')
  SELF_Demux : Subsystem  Tag=demux/SelfPort  mask(PreScan Demux Block:){}
      mask help:
      | The SELF port shows (state) information of the actor itself. The outputs are position in the experiment's axis system and the GPS coordinates, and the object's absolute velocity and compass heading.
      |
      | For more information, please click Help.
      settings: DeleteFcn=PreScanBlockDeleteFcn;
      mask Help: eval('openHelp(462)')
      mask Display:
      | port_label('output',1,'x [m]')
      | port_label('output',2,'y [m]')
      | port_label('output',3,'z [m]','texmode','on')
      | port_label('output',4,'Rotx [deg]','texmode','on')
      | port_label('output',5,'Roty [deg]','texmode','on')
      | port_label('output',6,'Rotz [deg]','texmode','on')
      | port_label('output',7,'GPS lat [deg]','texmode','on')
      | port_label('output',8,'GPS long [deg]','texmode','on')
      | port_label('output',9,'GPS alt [m]','texmode','on')
      | port_label('output',10,'Velocity [m/s]')
      | port_label('output',11,'Heading [deg]')
      | port_label('output',12,'Yaw rate [deg/s]')
  STATE_Audi_A8_4_rc : RateTransition  Tag=mux_rc/StatePort  OutPortSampleTimeOpt=Inherit
  Terminator_{1..12} (12 alike) : Terminator
  VISUColorRegion_Exterior_Mux : Subsystem  Tag=mux/MuxColorRegion  LoadFcn=load PrescanColorData  mask(PreScan User Interface: VisuTextureColor){}
      mask help:
      | The VisuTextureColor block provides a way to adapt the color of a vehicle.
      |
      | For more information, please click Help.
      settings: DeleteFcn=PreScanBlockDeleteFcn;
      mask Help: eval('openHelp(230)')
  STATE_Audi_A8_4_bus : Outport  Tag=outport/StatePort  OutDataTypeStr=Bus: PRESCAN_STATEACTUATORDATA  PortDimensions=1  SampleTime=1/100
  VISUColorRegion_Exterior_Audi_A8_4 : Outport  Tag=outport/ColorRegion  Port=2  OutDataTypeStr=Bus: PRESCAN_COLOR_DATA  PortDimensions=1  SampleTime=1/100
  wires:
  STATE_Audi_A8_4_rc/1 -> STATE_Audi_A8_4_bus/1
  SELF_Audi_A8_4/1 -> SELF_Demux/1(SELF)
  VISUColorRegion_Exterior_Mux/1(ColorRegion) -> VISUColorRegion_Exterior_Audi_A8_4/1
  ColorRegion_Exterior_color/1 -> VISUColorRegion_Exterior_Mux/1(RGB [-,-,-])
  Dynamics_Empty/1(State) -> STATE_Audi_A8_4_rc/1
  SELF_Demux/1(x [m]) -> Terminator_1/1
  SELF_Demux/2(y [m]) -> Terminator_2/1
  SELF_Demux/3(z [m]) -> Terminator_3/1
  SELF_Demux/4(rotx [deg]) -> Terminator_4/1
  SELF_Demux/5(roty [deg]) -> Terminator_5/1
  SELF_Demux/6(rotz [deg]) -> Terminator_6/1
  SELF_Demux/7(GPS lat [deg]) -> Terminator_7/1
  SELF_Demux/8(GPS long [deg]) -> Terminator_8/1
  SELF_Demux/9(GPS alt [m]) -> Terminator_9/1
  SELF_Demux/10(velocity [m/s]) -> Terminator_10/1
  SELF_Demux/11(heading [deg]) -> Terminator_11/1
  SELF_Demux/12(yaw rate [deg/s]) -> Terminator_12/1

== system ParkAssist_Scenario002_cs/Audi_A8_5 ==
  SELF_Audi_A8_5 : Inport  Tag=inport/SelfPort  OutDataTypeStr=Bus: PRESCAN_SELFSENSORDATA  PortDimensions=1  SampleTime=1/100  BusOutputAsStruct=on
  Dynamics_Empty : Subsystem  Tag=Dynamics_Empty
      mask Help: eval('openHelp(202)')
      mask Display: port_label('output', 1, 'State');text(0,0,' Empty\n')
  SELF_Demux : Subsystem  Tag=demux/SelfPort  mask(PreScan Demux Block:){}
      mask help:
      | The SELF port shows (state) information of the actor itself. The outputs are position in the experiment's axis system and the GPS coordinates, and the object's absolute velocity and compass heading.
      |
      | For more information, please click Help.
      settings: DeleteFcn=PreScanBlockDeleteFcn;
      mask Help: eval('openHelp(462)')
      mask Display:
      | port_label('output',1,'x [m]')
      | port_label('output',2,'y [m]')
      | port_label('output',3,'z [m]','texmode','on')
      | port_label('output',4,'Rotx [deg]','texmode','on')
      | port_label('output',5,'Roty [deg]','texmode','on')
      | port_label('output',6,'Rotz [deg]','texmode','on')
      | port_label('output',7,'GPS lat [deg]','texmode','on')
      | port_label('output',8,'GPS long [deg]','texmode','on')
      | port_label('output',9,'GPS alt [m]','texmode','on')
      | port_label('output',10,'Velocity [m/s]')
      | port_label('output',11,'Heading [deg]')
      | port_label('output',12,'Yaw rate [deg/s]')
  STATE_Audi_A8_5_rc : RateTransition  Tag=mux_rc/StatePort  OutPortSampleTimeOpt=Inherit
  Terminator_{1..12} (12 alike) : Terminator
  STATE_Audi_A8_5_bus : Outport  Tag=outport/StatePort  OutDataTypeStr=Bus: PRESCAN_STATEACTUATORDATA  PortDimensions=1  SampleTime=1/100
  wires:
  STATE_Audi_A8_5_rc/1 -> STATE_Audi_A8_5_bus/1
  SELF_Audi_A8_5/1 -> SELF_Demux/1(SELF)
  Dynamics_Empty/1(State) -> STATE_Audi_A8_5_rc/1
  SELF_Demux/1(x [m]) -> Terminator_1/1
  SELF_Demux/2(y [m]) -> Terminator_2/1
  SELF_Demux/3(z [m]) -> Terminator_3/1
  SELF_Demux/4(rotx [deg]) -> Terminator_4/1
  SELF_Demux/5(roty [deg]) -> Terminator_5/1
  SELF_Demux/6(rotz [deg]) -> Terminator_6/1
  SELF_Demux/7(GPS lat [deg]) -> Terminator_7/1
  SELF_Demux/8(GPS long [deg]) -> Terminator_8/1
  SELF_Demux/9(GPS alt [m]) -> Terminator_9/1
  SELF_Demux/10(velocity [m/s]) -> Terminator_10/1
  SELF_Demux/11(heading [deg]) -> Terminator_11/1
  SELF_Demux/12(yaw rate [deg/s]) -> Terminator_12/1

== system ParkAssist_Scenario002_cs/Audi_A8_9 ==
  SELF_Audi_A8_9 : Inport  Tag=inport/SelfPort  OutDataTypeStr=Bus: PRESCAN_SELFSENSORDATA  PortDimensions=1  SampleTime=1/100  BusOutputAsStruct=on
  ColorRegion_Exterior_color : Constant  Tag=VisuLightConst  Value=[192 192 192]
  Dynamics_Empty : Subsystem  Tag=Dynamics_Empty
      mask Help: eval('openHelp(202)')
      mask Display: port_label('output', 1, 'State');text(0,0,' Empty\n')
  SELF_Demux : Subsystem  Tag=demux/SelfPort  mask(PreScan Demux Block:){}
      mask help:
      | The SELF port shows (state) information of the actor itself. The outputs are position in the experiment's axis system and the GPS coordinates, and the object's absolute velocity and compass heading.
      |
      | For more information, please click Help.
      settings: DeleteFcn=PreScanBlockDeleteFcn;
      mask Help: eval('openHelp(462)')
      mask Display:
      | port_label('output',1,'x [m]')
      | port_label('output',2,'y [m]')
      | port_label('output',3,'z [m]','texmode','on')
      | port_label('output',4,'Rotx [deg]','texmode','on')
      | port_label('output',5,'Roty [deg]','texmode','on')
      | port_label('output',6,'Rotz [deg]','texmode','on')
      | port_label('output',7,'GPS lat [deg]','texmode','on')
      | port_label('output',8,'GPS long [deg]','texmode','on')
      | port_label('output',9,'GPS alt [m]','texmode','on')
      | port_label('output',10,'Velocity [m/s]')
      | port_label('output',11,'Heading [deg]')
      | port_label('output',12,'Yaw rate [deg/s]')
  STATE_Audi_A8_9_rc : RateTransition  Tag=mux_rc/StatePort  OutPortSampleTimeOpt=Inherit
  Terminator_{1..12} (12 alike) : Terminator
  VISUColorRegion_Exterior_Mux : Subsystem  Tag=mux/MuxColorRegion  LoadFcn=load PrescanColorData  mask(PreScan User Interface: VisuTextureColor){}
      mask help:
      | The VisuTextureColor block provides a way to adapt the color of a vehicle.
      |
      | For more information, please click Help.
      settings: DeleteFcn=PreScanBlockDeleteFcn;
      mask Help: eval('openHelp(230)')
  STATE_Audi_A8_9_bus : Outport  Tag=outport/StatePort  OutDataTypeStr=Bus: PRESCAN_STATEACTUATORDATA  PortDimensions=1  SampleTime=1/100
  VISUColorRegion_Exterior_Audi_A8_9 : Outport  Tag=outport/ColorRegion  Port=2  OutDataTypeStr=Bus: PRESCAN_COLOR_DATA  PortDimensions=1  SampleTime=1/100
  wires:
  STATE_Audi_A8_9_rc/1 -> STATE_Audi_A8_9_bus/1
  SELF_Audi_A8_9/1 -> SELF_Demux/1(SELF)
  VISUColorRegion_Exterior_Mux/1(ColorRegion) -> VISUColorRegion_Exterior_Audi_A8_9/1
  ColorRegion_Exterior_color/1 -> VISUColorRegion_Exterior_Mux/1(RGB [-,-,-])
  Dynamics_Empty/1(State) -> STATE_Audi_A8_9_rc/1
  SELF_Demux/1(x [m]) -> Terminator_1/1
  SELF_Demux/2(y [m]) -> Terminator_2/1
  SELF_Demux/3(z [m]) -> Terminator_3/1
  SELF_Demux/4(rotx [deg]) -> Terminator_4/1
  SELF_Demux/5(roty [deg]) -> Terminator_5/1
  SELF_Demux/6(rotz [deg]) -> Terminator_6/1
  SELF_Demux/7(GPS lat [deg]) -> Terminator_7/1
  SELF_Demux/8(GPS long [deg]) -> Terminator_8/1
  SELF_Demux/9(GPS alt [m]) -> Terminator_9/1
  SELF_Demux/10(velocity [m/s]) -> Terminator_10/1
  SELF_Demux/11(heading [deg]) -> Terminator_11/1
  SELF_Demux/12(yaw rate [deg/s]) -> Terminator_12/1

== system ParkAssist_Scenario002_cs/BMW_X5_1 ==
  SELF_BMW_X5_1 : Inport  Tag=inport/SelfPort  OutDataTypeStr=Bus: PRESCAN_SELFSENSORDATA  PortDimensions=1  SampleTime=1/100  BusOutputAsStruct=on
  Dynamics_Empty : Subsystem  Tag=Dynamics_Empty
      mask Help: eval('openHelp(202)')
      mask Display: port_label('output', 1, 'State');text(0,0,' Empty\n')
  SELF_Demux : Subsystem  Tag=demux/SelfPort  mask(PreScan Demux Block:){}
      mask help:
      | The SELF port shows (state) information of the actor itself. The outputs are position in the experiment's axis system and the GPS coordinates, and the object's absolute velocity and compass heading.
      |
      | For more information, please click Help.
      settings: DeleteFcn=PreScanBlockDeleteFcn;
      mask Help: eval('openHelp(462)')
      mask Display:
      | port_label('output',1,'x [m]')
      | port_label('output',2,'y [m]')
      | port_label('output',3,'z [m]','texmode','on')
      | port_label('output',4,'Rotx [deg]','texmode','on')
      | port_label('output',5,'Roty [deg]','texmode','on')
      | port_label('output',6,'Rotz [deg]','texmode','on')
      | port_label('output',7,'GPS lat [deg]','texmode','on')
      | port_label('output',8,'GPS long [deg]','texmode','on')
      | port_label('output',9,'GPS alt [m]','texmode','on')
      | port_label('output',10,'Velocity [m/s]')
      | port_label('output',11,'Heading [deg]')
      | port_label('output',12,'Yaw rate [deg/s]')
  STATE_BMW_X5_1_rc : RateTransition  Tag=mux_rc/StatePort  OutPortSampleTimeOpt=Inherit
  Terminator_{1..12} (12 alike) : Terminator
  STATE_BMW_X5_1_bus : Outport  Tag=outport/StatePort  OutDataTypeStr=Bus: PRESCAN_STATEACTUATORDATA  PortDimensions=1  SampleTime=1/100
  wires:
  STATE_BMW_X5_1_rc/1 -> STATE_BMW_X5_1_bus/1
  SELF_BMW_X5_1/1 -> SELF_Demux/1(SELF)
  Dynamics_Empty/1(State) -> STATE_BMW_X5_1_rc/1
  SELF_Demux/1(x [m]) -> Terminator_1/1
  SELF_Demux/2(y [m]) -> Terminator_2/1
  SELF_Demux/3(z [m]) -> Terminator_3/1
  SELF_Demux/4(rotx [deg]) -> Terminator_4/1
  SELF_Demux/5(roty [deg]) -> Terminator_5/1
  SELF_Demux/6(rotz [deg]) -> Terminator_6/1
  SELF_Demux/7(GPS lat [deg]) -> Terminator_7/1
  SELF_Demux/8(GPS long [deg]) -> Terminator_8/1
  SELF_Demux/9(GPS alt [m]) -> Terminator_9/1
  SELF_Demux/10(velocity [m/s]) -> Terminator_10/1
  SELF_Demux/11(heading [deg]) -> Terminator_11/1
  SELF_Demux/12(yaw rate [deg/s]) -> Terminator_12/1
